simulink model "downlink_4c2t"  (Simulink 8.7)
settings: Solver=VariableStepDiscrete  StartTime=0.0  StopTime=DUC_LINEUP_param.endTime  RelTol=1e-3
PreLoadFcn:
  | % Run the setup script when the model is opened
  | setup_downlink_4c2t;
InitFcn:
  | % Run the setup script again just before the
  | % model is run, so that any updates made
  | % after opening are applied.
  | setup_downlink_4c2t;
  | 
  | %% DSPBuilder Start
  | alt_dspbuilder_update_model(bdroot)
  | %% DSPBuilder End
values from neighbouring files (symbols this model uses):
  LUTS_DPD_CLIP =     [downlink_4c2t_dpd_clip.mat]
  PulsExtention = 128    [setup_downlink_4c2t.m]
  StartAddress1 = Iter1_Param.BaseAddr + 3200    [setup_downlink_4c2t.m]
  StartAddress2 = StartAddress1+1024    [setup_downlink_4c2t.m]
  win = [w(1:PulsExtention) ones(1,Iter0_Param.pulseLen) w(PulsExtention+1:end)]    [setup_downlink_4c2t.m]
undefined symbols (not defined in the file or in its folder): AdvDSPBChannelOutDisplay, AdvDSPBDMemDisplay, dpoly, dspba_ChannelInVis, dspba_ChannelOutVis, dspba_internal_get_channel_ports, dspba_internal_get_demux_ports, DUC_LINEUP_param, evalAionMaskParam, iq_width, Iter0_Param, latency, primtype, REG, UseDontCare, value
undefined symbols (not defined in the file): cfr0_id, cfr_Params0, cfr_Params1, clock_rate, REG_dut_id_addr
libraries: DSPBAPrim x1438, DSPBAControl x77, DSPBAModelBus x71, DSPBABase x40, downlink_4c2t_foldingcfr_3firs_lib x26, DSPBAUtilities x8, downlink_4c2t_lib x4, downlink_4c2t_cordic_lib x2, downlink_4c2t_dpd_clipper x2, DSPBAFilters x2, DSPBAWaveformSynth x2, downlink_4c2t_lduc_lib x1
(part 1 of 17)
Description:
  | DSP Builder Advanced Template for Template Design implementing ModelIP designs
settings Model: Creator=mjervis  LastModifiedBy=5g
settings DataIOCC: SignalLoggingSaveFormat=ModelDataLogs
settings OptimizationCC: ExpressionDepthLimit=2147483647
settings DebuggingCC: SolverPrmCheckMsg=warning  InheritedTsInSrcMsg=none  IntegerOverflowMsg=none  FcnCallInpInsideContextMsg=UseLocalSettings  StateNameClashWarn=warning  IntegerSaturationMsg=none
settings GRTTargetCC: CombineOutputUpdateFcns=off  GRTInterface=on

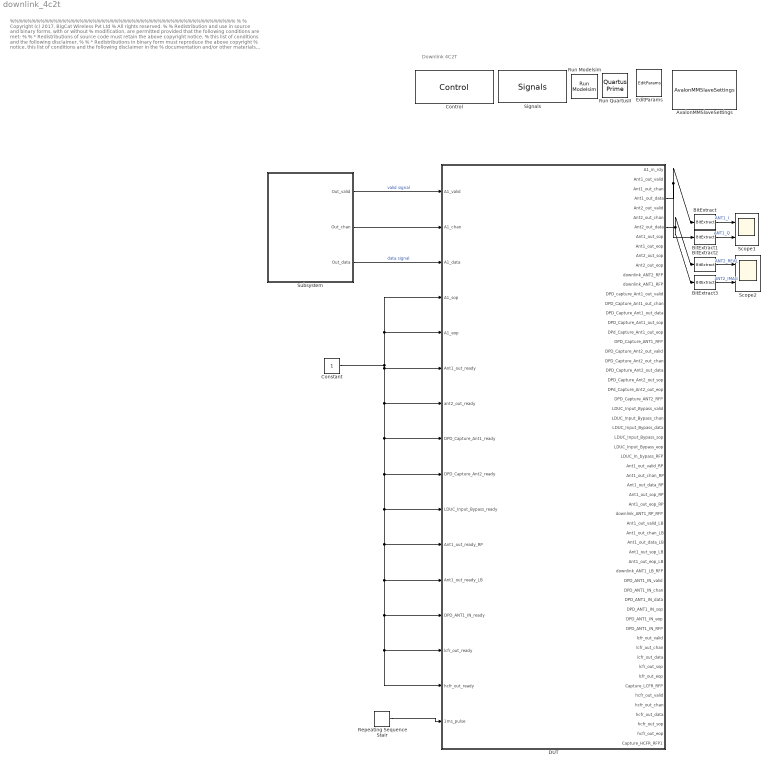
== system downlink_4c2t ==
  note: %%%%%%%%%%%%%%%%%%%%%%%%%%%%%%%%%%%%%%%%%%%%%%%%%%%%
      |  %
      |  % Copyright (c) 2017, BigCat Wireless Pvt Ltd
      |  % All rights reserved.
      |  %
      |  % Redistribution and use in source and binary forms, with or without
      |  % modification, are permitted provided that the following conditions are met:
      |  %
      |  %     * Redistributions of source code must retain the above copyright notice,
      |  %       this list of conditions and the following disclaimer.
      |  %
      |  %     * Redistributions in binary form must reproduce the above copyright
      |  %       notice, this list of conditions and the following disclaimer in the
      |  %       documentation and/or other materials provided with the distribution.
      |  %
      |  %     * Neither the name of the copyright holder nor the names of its contributors
      |  %       may be used to endorse or promote products derived from this software
      |  %       without specific prior written permission.
      |  %
      |  %
      |  %
      |  % THIS SOFTWARE IS PROVIDED BY THE COPYRIGHT HOLDERS AND CONTRIBUTORS "AS IS"
      |  % AND ANY EXPRESS OR IMPLIED WARRANTIES, INCLUDING, BUT NOT LIMITED TO, THE
      |  % IMPLIED WARRANTIES OF MERCHANTABILITY AND FITNESS FOR A PARTICULAR PURPOSE ARE
      |  % DISCLAIMED. IN NO EVENT SHALL THE COPYRIGHT HOLDER OR CONTRIBUTORS BE LIABLE
      |  % FOR ANY DIRECT, INDIRECT, INCIDENTAL, SPECIAL, EXEMPLARY, OR CONSEQUENTIAL
      |  % DAMAGES (INCLUDING, BUT NOT LIMITED TO, PROCUREMENT OF SUBSTITUTE GOODS OR
      |  % SERVICES; LOSS OF USE, DATA, OR PROFITS; OR BUSINESS INTERRUPTION) HOWEVER
      |  % CAUSED AND ON ANY THEORY OF LIABILITY, WHETHER IN CONTRACT, STRICT LIABILITY,
      |  % OR TORT (INCLUDING NEGLIGENCE OR OTHERWISE) ARISING IN ANY WAY OUT OF THE USE
      |  % OF THIS SOFTWARE, EVEN IF ADVISED OF THE POSSIBILITY OF SUCH DAMAGE.
      |  %
      |   %%%%%%%%%%%%%%%%%%%%%%%%%%%%%%%%%%%%%%%%%%%%%%%%%%%%%
  note: Downlink 4C2T
  AvalonMMSlaveSettings : DSPBABase/AvalonMMSlaveSettings
  BitExtract : DSPBAPrim/BitExtract  primtype=bitextract  nInputs=1  nOutputs=1  omode=Specify via dialog  otype=sfix(16)  scale=2^-15  rndmethod=Unbiased  factor=1  satmethod=Symmetric  shift_vec=[0 1 2 -1]  value=0  inPortNames=[' '; ' ';]  outPortNames=[' ']  dspbaimage=dspba_prim.jpg  text=fprintf('..%d', value);  style=Optimised  visibilities=8+1024  version=20090407
  BitExtract1 : DSPBAPrim/BitExtract  primtype=bitextract  nInputs=1  nOutputs=1  omode=Specify via dialog  otype=sfix(16)  scale=2^-15  rndmethod=Unbiased  factor=1  satmethod=Symmetric  shift_vec=[0 1 2 -1]  value=16  inPortNames=[' '; ' ';]  outPortNames=[' ']  dspbaimage=dspba_prim.jpg  text=fprintf('..%d', value);  style=Optimised  visibilities=8+1024  version=20090407
  BitExtract2 : DSPBAPrim/BitExtract  primtype=bitextract  nInputs=1  nOutputs=1  omode=Specify via dialog  otype=sfix(16)  scale=2^-15  rndmethod=Unbiased  factor=1  satmethod=Symmetric  shift_vec=[0 1 2 -1]  value=0  inPortNames=[' '; ' ';]  outPortNames=[' ']  dspbaimage=dspba_prim.jpg  text=fprintf('..%d', value);  style=Optimised  visibilities=8+1024  version=20090407
  BitExtract3 : DSPBAPrim/BitExtract  primtype=bitextract  nInputs=1  nOutputs=1  omode=Specify via dialog  otype=sfix(16)  scale=2^-15  rndmethod=Unbiased  factor=1  satmethod=Symmetric  shift_vec=[0 1 2 -1]  value=16  inPortNames=[' '; ' ';]  outPortNames=[' ']  dspbaimage=dspba_prim.jpg  text=fprintf('..%d', value);  style=Optimised  visibilities=8+1024  version=20090407
  Constant : Constant  OutDataTypeStr=boolean
  Control : DSPBABase/Control  generate=on  language=VHDL  destination=./rtl  destination_gui=./rtl  make_full_path=off  path_is_relative=on  autotestbench=off  signaldepth=2  coveragetestbench=off  logs=off  spacewidth=2  spacenum=1  addrwidth=14  datawidth=32  dataendian=Big Endian  hierarchicalnames=off  ramThresholdBits=-1  distRamThresholdBits=-1  mlabThresholdBits=-1  hardMultiplierThresholdLuts=-1  version=20090407  errorOnChanMismatch=1  errorOnGPIOMismatch=0  importModelsimResults=0  cycleAccurate=off  reinterpretCastMult=off  paramFile=downlink_4c2t_params.xml
  DUT : Subsystem
  EditParams : DSPBABase/EditParams  version=20090407
  Repeating Sequence Stair : simulink/Sources/Repeating Sequence Stair  OutValues=[zeros(1,1000) 1 1 1 1].'  tsamp=-1  OutMin=[]  OutMax=[]  OutDataTypeStr=fixdt('boolean')  OutputDataTypeScalingMode=Specify via dialog  OutDataType=fixdt('boolean')  ConRadixGroup=Best Precision: Vector-wise  OutScaling=[]
  Run Modelsim : DSPBABase/Run Modelsim  version=20090407
  "Run QuartusII " : DSPBABase/Quartus Prime  version=20090407
  Scope1 : Scope  NumInputPorts=2
  Scope2 : Scope  NumInputPorts=2
  Signals : DSPBABase/Signals  clk=clk  freq=DUC_LINEUP_param.ClockRate  margin=DUC_LINEUP_param.ClockMargin  rst=areset  rstactive=High  bus=bus  enbusclock=on  busfreq=61.44  bussync=on  version=20090407
  Subsystem : Subsystem
  wires:
  Subsystem/3(Out_data) -> DUT/3(A1_data)  "data signal"
  Subsystem/1(Out_valid) -> DUT/1(A1_valid)  "valid signal"
  Subsystem/2(Out_chan) -> DUT/2(A1_chan)
  Constant/1 -> DUT/8(DPD_Capture_Ant1_ready), DUT/9(DPD_Capture_Ant2_ready), DUT/10(LDUC_Input_Bypass_ready), DUT/11(Ant1_out_ready_RP), DUT/12(Ant1_out_ready_LB), DUT/14(lcfr_out_ready), DUT/15(hcfr_out_ready), DUT/13(DPD_ANT1_IN_ready), DUT/7(ant2_out_ready), DUT/6(Ant1_out_ready), DUT/4(A1_sop), DUT/5(A1_eop)
  DUT/7(Ant2_out_data) -> BitExtract2/1, BitExtract3/1
  BitExtract/1 -> Scope1/1  "ANT1_I"
  BitExtract1/1 -> Scope1/2  "ANT1_Q"
  BitExtract2/1 -> Scope2/1  "ANT2_REAL"
  BitExtract3/1 -> Scope2/2  "ANT2_IMAG"
  Repeating Sequence Stair/1 -> DUT/16(1ms_pulse)
  DUT/4(Ant1_out_data) -> BitExtract1/1, BitExtract/1

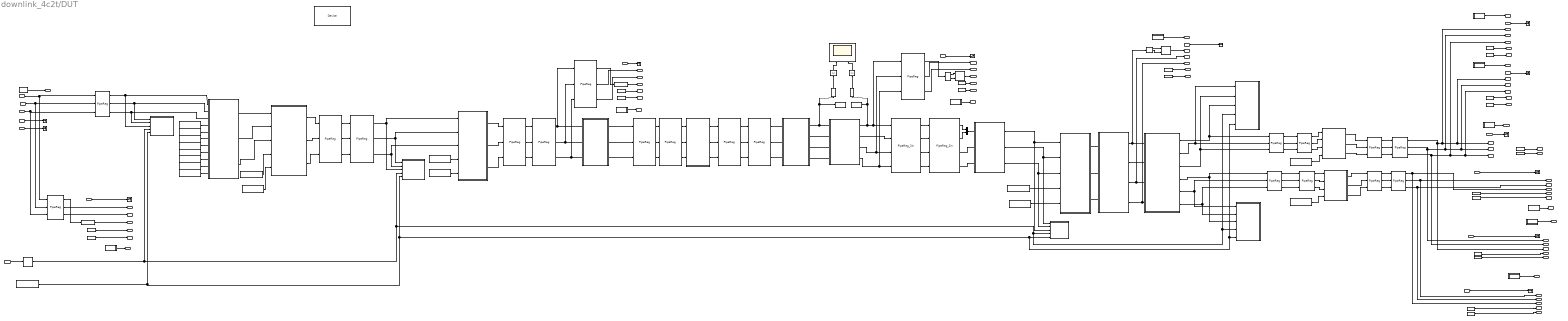
== system downlink_4c2t/DUT ==
  A1_valid : Inport
  A1_chan : Inport  Port=2
  A1_data : Inport  Port=3
  A1_sop : Inport  Port=4
  A1_eop : Inport  Port=5
  Ant1_out_ready : Inport  Port=6
  ant2_out_ready : Inport  Port=7
  DPD_Capture_Ant1_ready : Inport  Port=8
  DPD_Capture_Ant2_ready : Inport  Port=9
  LDUC_Input_Bypass_ready : Inport  Port=10
  Ant1_out_ready_RP : Inport  Port=11
  Ant1_out_ready_LB : Inport  Port=12
  DPD_ANT1_IN_ready : Inport  Port=13
  lcfr_out_ready : Inport  Port=14
  hcfr_out_ready : Inport  Port=15
  1ms_pulse : Inport  Port=16
  ANT1_rfp : Subsystem
  ANT2_rfp : Subsystem
  Abs2 : Abs
  Abs3 : Abs
  BLIND_CFR : Subsystem
  BitCombine : DSPBAPrim/BitCombine  primtype=bitcombine  nInputs=2  nOutputs=1  omode=Inherit via internal rule  otype=sfix(16)  scale=2^-15  rndmethod=Unbiased  factor=1  satmethod=Symmetric  shift_vec=[0 1 2 -1]  value=0  inPortNames=['l'; 'h';]  outPortNames=[' ']  dspbaimage=dspba_prim.jpg  text=fprintf('[h,l]');  style=Optimised  visibilities=8+2  version=20090407
  BitCombine1 : DSPBAPrim/BitCombine  primtype=bitcombine  nInputs=2  nOutputs=1  omode=Inherit via internal rule  otype=sfix(16)  scale=2^-15  rndmethod=Unbiased  factor=1  satmethod=Symmetric  shift_vec=[0 1 2 -1]  value=0  inPortNames=['l'; 'h';]  outPortNames=[' ']  dspbaimage=dspba_prim.jpg  text=fprintf('[h,l]');  style=Optimised  visibilities=8+2  version=20090407
  COMPLEX_REAL : Subsystem
  Complex to Real-Imag : ComplexToRealImag
  Complex to Real-Imag1 : ComplexToRealImag
  Const1 : DSPBAPrim/Const  primtype=const  nInputs=0  nOutputs=1  omode=boolean  otype=sfix(16)  scale=2^-15  rndmethod=Unbiased  factor=1  satmethod=Symmetric  shift_vec=[0 1 2 -1]  value=1  inPortNames=['+'; '+';]  outPortNames=[' ']  dspbaimage=dspba_prim.jpg  text=fprintf('%s', num2str(value));  style=Optimised  visibilities=8 + 1024  floatPrecision=float32_m23  version=20120820
  Const{2..17,19,30} (18 alike) : DSPBAPrim/Const  primtype=const  nInputs=0  nOutputs=1  omode=Inherit via internal rule  otype=sfix(16)  scale=2^-15  rndmethod=Unbiased  factor=1  satmethod=Symmetric  shift_vec=[0 1 2 -1]  value=1  inPortNames=['+'; '+';]  outPortNames=[' ']  dspbaimage=dspba_prim.jpg  text=fprintf('%s', num2str(value));  style=Optimised  visibilities=8 + 1024  floatPrecision=float32_m23  version=20120820
  Const18 : DSPBAPrim/Const  primtype=const  nInputs=0  nOutputs=1  omode=boolean  otype=sfix(16)  scale=2^-15  rndmethod=Unbiased  factor=1  satmethod=Symmetric  shift_vec=[0 1 2 -1]  value=1  inPortNames=['+'; '+';]  outPortNames=[' ']  dspbaimage=dspba_prim.jpg  text=fprintf('%s', num2str(value));  style=Optimised  visibilities=8 + 1024  floatPrecision=float32_m23  version=20120820
  Const29 : DSPBAPrim/Const  primtype=const  nInputs=0  nOutputs=1  omode=boolean  otype=sfix(16)  scale=2^-15  rndmethod=Unbiased  factor=1  satmethod=Symmetric  shift_vec=[0 1 2 -1]  value=1  inPortNames=['+'; '+';]  outPortNames=[' ']  dspbaimage=dspba_prim.jpg  text=fprintf('%s', num2str(value));  style=Optimised  visibilities=8 + 1024  floatPrecision=float32_m23  version=20120820
  Convert1 : DSPBAPrim/Convert  primtype=convert  nInputs=1  nOutputs=1  omode=Specify via dialog  otype=sfix(32)  scale=2^-31  rndmethod=Unbiased  factor=1  satmethod=None  shift_vec=[0 1 2 -1]  value=round([0:255]/17)  inPortNames=[' '; ' ';]  outPortNames=[' '; 'c']  dspbaimage=dspba_prim.jpg  text=fprintf('convert');  style=Optimised  visibilities=8+64+256+2^17  clipdetect=off  floatPrecision=float32_m23  advOptions=[]  version=20130211
  Convert2 : DSPBAPrim/Convert  primtype=convert  nInputs=1  nOutputs=1  omode=Specify via dialog  otype=sfix(32)  scale=2^-31  rndmethod=Unbiased  factor=1  satmethod=None  shift_vec=[0 1 2 -1]  value=round([0:255]/17)  inPortNames=[' '; ' ';]  outPortNames=[' '; 'c']  dspbaimage=dspba_prim.jpg  text=fprintf('convert');  style=Optimised  visibilities=8+64+256+2^17  clipdetect=off  floatPrecision=float32_m23  advOptions=[]  version=20130211
  DPD : Subsystem
  DPD1_CLIPPER : Subsystem
  DPD2_CLIPPER : Subsystem
  DPD_ANT1_IN_rfp : Subsystem
  DUC_DPD1_OUT_PM : Subsystem
  DUC_DPD2_OUT_PM : Subsystem
  DUC_DPD_IN_PM : Subsystem
  DUC_IN_PM : Subsystem
  DUC_SUMMER_PM : Subsystem
  Data Type Conversion2 : DataTypeConversion  OutDataTypeStr=double
  Data Type Conversion4 : DataTypeConversion  OutDataTypeStr=double
  Device : DSPBABase/Device  family=Arria 10  deviceMember=Arria 10  stratix4device=Stratix IV GX  hardcopy4device=HardCopy IV E  stratix5device=Stratix V GX  device=10AS066N3F40E2SGE2  speed=2  stratixSpeed=-5  stratix2Speed=-3  stratix3Speed=-3  stratix4gxSpeed=-2  stratix4gtSpeed=-1  cyclone2Speed=-6  cyclone3Speed=-7  arria2Speed=-4  cyclone4eSpeed=-8  stratix5Speed=-3  arria5Speed=-4  arriaSpeed=-6  cyclone3lsSpeed=-7  cyclone5Speed=-6  arria2gzSpeed=-3  nightFurySpeed=-2  ecp2Speed=-7  hardcopycompat=off  version=20140217  max10flashmode=off  max10nomeminit=off
  Downlink_ANT1_LB_rfp : Subsystem
  Downlink_ANT1_RP_rfp : Subsystem
  Gain_dpd_input : Subsystem
  Gain_duc_input : Subsystem
  Gain_summer : Subsystem
  HDUC_STG1 : Subsystem
  HDUC_STG2 : Subsystem
  LDUC : Subsystem
  Mux : Mux  Inputs=2
  PipeReg_2in : downlink_4c2t_foldingcfr_3firs_lib/PipeReg_2in  NPipe=2  Clock_Margin=DUC_LINEUP_param.ClockMargin
      link override ChannelOut: value=2  packetBeginEnabled=off  latency=2
  PipeReg_2in1 : downlink_4c2t_foldingcfr_3firs_lib/PipeReg_2in  NPipe=2  Clock_Margin=DUC_LINEUP_param.ClockMargin
      link override ChannelOut: value=2  packetBeginEnabled=off  latency=2
  PipeReg_CM_HDUC_R1 : downlink_4c2t_foldingcfr_3firs_lib/PipeReg  NPipe=2  Clock_Margin=DUC_LINEUP_param.ClockMargin
      link override ChannelOut: latency=2  value=1  packetBeginEnabled=off
  PipeReg_HDCU2_RC1 : downlink_4c2t_foldingcfr_3firs_lib/PipeReg  NPipe=2  Clock_Margin=DUC_LINEUP_param.ClockMargin
      link override ChannelOut: latency=2  value=1  packetBeginEnabled=off
  PipeReg_HDCU2_RC_L1 : downlink_4c2t_foldingcfr_3firs_lib/PipeReg  NPipe=2  Clock_Margin=DUC_LINEUP_param.ClockMargin
      link override ChannelOut: latency=2  value=1  packetBeginEnabled=off
  PipeReg_HDUC2_RC_L1 : downlink_4c2t_foldingcfr_3firs_lib/PipeReg  NPipe=2  Clock_Margin=DUC_LINEUP_param.ClockMargin
      link override ChannelOut: latency=2  value=1  packetBeginEnabled=off
  PipeReg_HDUC_RC_L : downlink_4c2t_foldingcfr_3firs_lib/PipeReg  NPipe=2  Clock_Margin=DUC_LINEUP_param.ClockMargin
      link override ChannelOut: value=1  packetBeginEnabled=off  latency=2
  PipeReg_HDUC_RC_R : downlink_4c2t_foldingcfr_3firs_lib/PipeReg  NPipe=2  Clock_Margin=DUC_LINEUP_param.ClockMargin
      link override ChannelOut: latency=2  value=1  packetBeginEnabled=off
  PipeReg_avln_avln_R : downlink_4c2t_foldingcfr_3firs_lib/PipeReg  NPipe=6  Clock_Margin=DUC_LINEUP_param.ClockMargin
      link override ChannelOut: latency=6  value=1  packetBeginEnabled=off
  PipeReg_dpd1clip_avln_L : downlink_4c2t_foldingcfr_3firs_lib/PipeReg  NPipe=2  Clock_Margin=DUC_LINEUP_param.ClockMargin
      link override ChannelOut: latency=2  value=1  packetBeginEnabled=off
  PipeReg_dpd1clip_avln_R : downlink_4c2t_foldingcfr_3firs_lib/PipeReg  NPipe=2  Clock_Margin=DUC_LINEUP_param.ClockMargin
      link override ChannelOut: latency=2  value=1  packetBeginEnabled=off
  PipeReg_dpd1gain_dpd1clip_L : downlink_4c2t_foldingcfr_3firs_lib/PipeReg  NPipe=2  Clock_Margin=DUC_LINEUP_param.ClockMargin
      link override ChannelOut: latency=2  value=1  packetBeginEnabled=off
  PipeReg_dpd1gain_dpd1clip_R : downlink_4c2t_foldingcfr_3firs_lib/PipeReg  NPipe=2  Clock_Margin=DUC_LINEUP_param.ClockMargin
      link override ChannelOut: latency=2  value=1  packetBeginEnabled=off
  PipeReg_dpd2clip_avln_L : downlink_4c2t_foldingcfr_3firs_lib/PipeReg  NPipe=2  Clock_Margin=DUC_LINEUP_param.ClockMargin
      link override ChannelOut: latency=2  value=1  packetBeginEnabled=off
  PipeReg_dpd2clip_avln_R : downlink_4c2t_foldingcfr_3firs_lib/PipeReg  NPipe=2  Clock_Margin=DUC_LINEUP_param.ClockMargin
      link override ChannelOut: latency=2  value=1  packetBeginEnabled=off
  PipeReg_dpd2gain_dpd2clip_L : downlink_4c2t_foldingcfr_3firs_lib/PipeReg  NPipe=2  Clock_Margin=DUC_LINEUP_param.ClockMargin
      link override ChannelOut: latency=2  value=1  packetBeginEnabled=off
  PipeReg_dpd2gain_dpd2clip_R : downlink_4c2t_foldingcfr_3firs_lib/PipeReg  NPipe=2  Clock_Margin=DUC_LINEUP_param.ClockMargin
      link override ChannelOut: latency=2  value=1  packetBeginEnabled=off
  PipeReg_lduc_RC_L : downlink_4c2t_foldingcfr_3firs_lib/PipeReg  NPipe=2  Clock_Margin=DUC_LINEUP_param.ClockMargin
      link override ChannelOut: latency=2  value=1  packetBeginEnabled=off
  PipeReg_lduc_RC_R : downlink_4c2t_foldingcfr_3firs_lib/PipeReg  NPipe=2  Clock_Margin=DUC_LINEUP_param.ClockMargin
      link override ChannelOut: latency=2  value=1  packetBeginEnabled=off
  PipeReg_lduc_hduc1_L : downlink_4c2t_foldingcfr_3firs_lib/PipeReg  NPipe=2  Clock_Margin=DUC_LINEUP_param.ClockMargin
      link override ChannelOut: latency=2  value=1  packetBeginEnabled=off
  PipeReg_lduc_hduc1_L2 : downlink_4c2t_foldingcfr_3firs_lib/PipeReg  NPipe=6  Clock_Margin=DUC_LINEUP_param.ClockMargin
      link override ChannelOut: latency=6  value=1  packetBeginEnabled=off
  PipeReg_lduc_hduc1_R : downlink_4c2t_foldingcfr_3firs_lib/PipeReg  NPipe=2  Clock_Margin=DUC_LINEUP_param.ClockMargin
      link override ChannelOut: latency=2  value=1  packetBeginEnabled=off
  REAL_COMPLEX1 : Subsystem
  REAL_COMPLEX2 : Subsystem
  RegBit : DSPBAModelBus/RegBit  reg_name=Reg_busy_bit_addr  reg_rwmode=Read/Write  reg_lsb=0  reg_init=0  reg_desc=Reg_busy_bi will be stored here  reg_addr=9686  reg_desc0=0  reg_desc1=0  SampleTime=-1  version=20090407
  RegBit1 : DSPBAModelBus/RegBit  reg_name=DUC_LINEUP_param.A12xC_NCO.Sync  reg_rwmode=Read/Write  reg_lsb=0  reg_init=0  reg_desc=Description of what is stored in this field  reg_addr=768  reg_desc0=0  reg_desc1=0  SampleTime=1  version=20090407
  RegField : DSPBAModelBus/RegField  reg_name=Sum_shifter_addr  reg_rwmode=Read/Write  reg_msb=1  reg_lsb=0  reg_mode=Specify via dialog  reg_type=uint(2)  reg_scale=2^-0  reg_init=Sum_shifter_init_value  reg_desc=Sum_shifter_init_value will be stored  reg_modal=off  reg_desc0=0  reg_desc1=0  reg_desc2=0  reg_desc3=0  reg_desc4=0  reg_desc5=0  reg_desc6=0  reg_desc7=0  reg_addr=9643  SampleTime=-1  version=20090407
  RegField1 : DSPBAModelBus/RegField  reg_name=DPD1_CLIP_SCALE  reg_rwmode=Read/Write  reg_msb=0  reg_lsb=0  reg_mode=Specify via dialog  reg_type=ufix(1)  reg_scale=1  reg_init=DPD1_CLIP_INIT_VALUE  reg_desc=DPD1_CLIP_INIT_VALUE will be stored  reg_modal=off  reg_desc0=0  reg_desc1=0  reg_desc2=0  reg_desc3=0  reg_desc4=0  reg_desc5=0  reg_desc6=0  reg_desc7=0  reg_addr=9691  SampleTime=-1  version=20090407
  RegField10 : DSPBAModelBus/RegField  reg_name=ant1_summer_gain_addr  reg_rwmode=Read/Write  reg_msb=15  reg_lsb=0  reg_mode=Specify via dialog  reg_type=ufix(16)  reg_scale=2^-12  reg_init=ant1_summer_gain_init  reg_desc=ant1_summer_gain will be stored here  reg_modal=off  reg_desc0=0  reg_desc1=0  reg_desc2=0  reg_desc3=0  reg_desc4=0  reg_desc5=0  reg_desc6=0  reg_desc7=0  reg_addr=9624  SampleTime=-1  version=20090407
  RegField11 : DSPBAModelBus/RegField  reg_name=ant2_summer_gain_addr  reg_rwmode=Read/Write  reg_msb=15  reg_lsb=0  reg_mode=Specify via dialog  reg_type=ufix(16)  reg_scale=2^-12  reg_init=ant2_summer_gain_init  reg_desc=ant2_summer_gain will be stored here  reg_modal=off  reg_desc0=0  reg_desc1=0  reg_desc2=0  reg_desc3=0  reg_desc4=0  reg_desc5=0  reg_desc6=0  reg_desc7=0  reg_addr=9625  SampleTime=-1  version=20090407
  RegField12 : DSPBAModelBus/RegField  reg_name=dpd1_gain_addr  reg_rwmode=Read/Write  reg_msb=15  reg_lsb=0  reg_mode=Specify via dialog  reg_type=ufix(16)  reg_scale=2^-12  reg_init=dpd1_gain_init_value  reg_desc=dpd1_gain will be stored here  reg_modal=off  reg_desc0=0  reg_desc1=0  reg_desc2=0  reg_desc3=0  reg_desc4=0  reg_desc5=0  reg_desc6=0  reg_desc7=0  reg_addr=9626  SampleTime=-1  version=20090407
  RegField13 : DSPBAModelBus/RegField  reg_name=dpd2_gain_addr  reg_rwmode=Read/Write  reg_msb=15  reg_lsb=0  reg_mode=Specify via dialog  reg_type=ufix(16)  reg_scale=2^-12  reg_init=dpd2_gain_init_value  reg_desc=dpd2_gain will be stored here  reg_modal=off  reg_desc0=0  reg_desc1=0  reg_desc2=0  reg_desc3=0  reg_desc4=0  reg_desc5=0  reg_desc6=0  reg_desc7=0  reg_addr=9627  SampleTime=-1  version=20090407
  RegField14 : DSPBAModelBus/RegField  reg_name=DPD2_CLIP_SCALE  reg_rwmode=Read/Write  reg_msb=0  reg_lsb=0  reg_mode=Specify via dialog  reg_type=ufix(1)  reg_scale=1  reg_init=DPD2_CLIP_INIT_VALUE  reg_desc=DPD2_CLIP_INIT_VALUE will be stored  reg_modal=off  reg_desc0=0  reg_desc1=0  reg_desc2=0  reg_desc3=0  reg_desc4=0  reg_desc5=0  reg_desc6=0  reg_desc7=0  reg_addr=9692  SampleTime=-1  version=20090407
  RegField2 : DSPBAModelBus/RegField  reg_name=ant1_carr1_gain_addr  reg_rwmode=Read/Write  reg_msb=15  reg_lsb=0  reg_mode=Specify via dialog  reg_type=ufix(16)  reg_scale=2^-12  reg_init=ant1_carr1_gain_val_init  reg_desc=ant1_carr1_gain will be stored here  reg_modal=off  reg_desc0=0  reg_desc1=0  reg_desc2=0  reg_desc3=0  reg_desc4=0  reg_desc5=0  reg_desc6=0  reg_desc7=0  reg_addr=9616  SampleTime=-1  version=20090407
  RegField3 : DSPBAModelBus/RegField  reg_name=ant1_carr2_gain_addr  reg_rwmode=Read/Write  reg_msb=15  reg_lsb=0  reg_mode=Specify via dialog  reg_type=ufix(16)  reg_scale=2^-12  reg_init=ant1_carr2_gain_val_init  reg_desc=ant1_carr2_gain will be stored here  reg_modal=off  reg_desc0=0  reg_desc1=0  reg_desc2=0  reg_desc3=0  reg_desc4=0  reg_desc5=0  reg_desc6=0  reg_desc7=0  reg_addr=9617  SampleTime=-1  version=20090407
  RegField4 : DSPBAModelBus/RegField  reg_name=ant1_carr3_gain_addr  reg_rwmode=Read/Write  reg_msb=15  reg_lsb=0  reg_mode=Specify via dialog  reg_type=ufix(16)  reg_scale=2^-12  reg_init=ant1_carr3_gain_val_init  reg_desc=ant1_carr3_gain will be stored here  reg_modal=off  reg_desc0=0  reg_desc1=0  reg_desc2=0  reg_desc3=0  reg_desc4=0  reg_desc5=0  reg_desc6=0  reg_desc7=0  reg_addr=9618  SampleTime=-1  version=20090407
  RegField5 : DSPBAModelBus/RegField  reg_name=ant1_carr4_gain_addr  reg_rwmode=Read/Write  reg_msb=15  reg_lsb=0  reg_mode=Specify via dialog  reg_type=ufix(16)  reg_scale=2^-12  reg_init=ant1_carr4_gain_val_init  reg_desc=ant1_carr4_gain will be stored here  reg_modal=off  reg_desc0=0  reg_desc1=0  reg_desc2=0  reg_desc3=0  reg_desc4=0  reg_desc5=0  reg_desc6=0  reg_desc7=0  reg_addr=9619  SampleTime=-1  version=20090407
  RegField6 : DSPBAModelBus/RegField  reg_name=ant2_carr1_gain_addr  reg_rwmode=Read/Write  reg_msb=15  reg_lsb=0  reg_mode=Specify via dialog  reg_type=ufix(16)  reg_scale=2^-12  reg_init=ant2_carr1_gain_val_init  reg_desc=ant2_carr1_gain will be stored here  reg_modal=off  reg_desc0=0  reg_desc1=0  reg_desc2=0  reg_desc3=0  reg_desc4=0  reg_desc5=0  reg_desc6=0  reg_desc7=0  reg_addr=9620  SampleTime=-1  version=20090407
  RegField7 : DSPBAModelBus/RegField  reg_name=ant2_carr2_gain_addr  reg_rwmode=Read/Write  reg_msb=15  reg_lsb=0  reg_mode=Specify via dialog  reg_type=ufix(16)  reg_scale=2^-12  reg_init=ant2_carr2_gain_val_init  reg_desc=ant2_carr2_gain will be stored here  reg_modal=off  reg_desc0=0  reg_desc1=0  reg_desc2=0  reg_desc3=0  reg_desc4=0  reg_desc5=0  reg_desc6=0  reg_desc7=0  reg_addr=9621  SampleTime=-1  version=20090407
  RegField8 : DSPBAModelBus/RegField  reg_name=ant2_carr3_gain_addr  reg_rwmode=Read/Write  reg_msb=15  reg_lsb=0  reg_mode=Specify via dialog  reg_type=ufix(16)  reg_scale=2^-12  reg_init=ant2_carr3_gain_val_init  reg_desc=ant2_carr3_gain will be stored here  reg_modal=off  reg_desc0=0  reg_desc1=0  reg_desc2=0  reg_desc3=0  reg_desc4=0  reg_desc5=0  reg_desc6=0  reg_desc7=0  reg_addr=9622  SampleTime=-1  version=20090407
  RegField9 : DSPBAModelBus/RegField  reg_name=ant2_carr4_gain_addr  reg_rwmode=Read/Write  reg_msb=15  reg_lsb=0  reg_mode=Specify via dialog  reg_type=ufix(16)  reg_scale=2^-12  reg_init=ant2_carr4_gain_val_init  reg_desc=ant2_carr4_gain will be stored here  reg_modal=off  reg_desc0=0  reg_desc1=0  reg_desc2=0  reg_desc3=0  reg_desc4=0  reg_desc5=0  reg_desc6=0  reg_desc7=0  reg_addr=9623  SampleTime=-1  version=20090407
  SampleDelay : DSPBAPrim/SampleDelay  primtype=sampdelay  nInputs=1  nOutputs=1  omode=Inherit via internal rule  otype=sfix(16)  scale=2^-15  rndmethod=Unbiased  factor=1  satmethod=Symmetric  shift_vec=[0 1 2 -1]  value=4  inPortNames=[' '; ' ';]  outPortNames=[' ']  dspbaimage=dspba_prim.jpg  text=dpoly(1, eye(1,value+1), 'z')  style=Optimised  visibilities=8 + 1024 + 2^17 + 2^18  flexible=off  slackgroup=0  augmented=0  version=20090407  advOptions=[]
  Scope1 : Scope  NumInputPorts=2
  Terminator{1..10,19..20} (12 alike) : Terminator
  To Workspace1 : ToWorkspace  VariableName=cfr_input  SaveFormat=Structure With Time  SampleTime=1
  To Workspace3 : ToWorkspace  VariableName=cfr_output  SaveFormat=Structure With Time  SampleTime=1
  dpd_ant1_out_rfp : Subsystem
  dpd_ant2_out_rfp : Subsystem
  lcfr_rfp : Subsystem
  lcfr_rfp1 : Subsystem
  lduc_bypass_rfp : Subsystem
  A1_in_rdy : Outport
  Ant1_out_valid : Outport  Port=2
  Ant1_out_chan : Outport  Port=3
  Ant1_out_data : Outport  Port=4
  Ant2_out_valid : Outport  Port=5
  Ant2_out_chan : Outport  Port=6
  Ant2_out_data : Outport  Port=7
  Ant1_out_sop : Outport  Port=8
  Ant1_out_eop : Outport  Port=9
  Ant2_out_sop : Outport  Port=10
  Ant2_out_eop : Outport  Port=11
  downlink_ANT2_RFP : Outport  Port=12
  downlink_ANT1_RFP : Outport  Port=13
  DPD_capture_Ant1_out_valid : Outport  Port=14
  DPD_Capture_Ant1_out_chan : Outport  Port=15
  DPD_Capture_Ant1_out_data : Outport  Port=16
  DPD_Capture_Ant1_out_sop : Outport  Port=17
  DPd_Capture_Ant1_out_eop : Outport  Port=18
  DPD_Capture_ANT1_RFP : Outport  Port=19
  DPD_Capture_Ant2_out_valid : Outport  Port=20
  DPD_Capture_Ant2_out_chan : Outport  Port=21
  DPD_Capture_Ant2_out_data : Outport  Port=22
  DPD_Capture_Ant2_out_sop : Outport  Port=23
  DPd_Capture_Ant2_out_eop : Outport  Port=24
  DPD_Capture_ANT2_RFP : Outport  Port=25
  LDUC_Input_Bypass_valid : Outport  Port=26
  LDUC_Input_Bypass_chan : Outport  Port=27
  LDUC_Input_Bypass_data : Outport  Port=28
  LDUC_Input_Bypass_sop : Outport  Port=29
  LDUC_Input_Bypass_eop : Outport  Port=30
  LDUC_In_bypass_RFP : Outport  Port=31
  Ant1_out_valid_RP : Outport  Port=32
  Ant1_out_chan_RP : Outport  Port=33
  Ant1_out_data_RP : Outport  Port=34
  Ant1_out_sop_RP : Outport  Port=35
  Ant1_out_eop_RP : Outport  Port=36
  downlink_ANT1_RP_RFP : Outport  Port=37
  Ant1_out_valid_LB : Outport  Port=38
  Ant1_out_chan_LB : Outport  Port=39
  Ant1_out_data_LB : Outport  Port=40
  Ant1_out_sop_LB : Outport  Port=41
  Ant1_out_eop_LB : Outport  Port=42
  downlink_ANT1_LB_RFP : Outport  Port=43
  DPD_ANT1_IN_valid : Outport  Port=44
  DPD_ANT1_IN_chan : Outport  Port=45
  DPD_ANT1_IN_data : Outport  Port=46
  DPD_ANT1_IN_sop : Outport  Port=47
  DPD_ANT1_IN_eop : Outport  Port=48
  DPD_ANT1_IN_RFP : Outport  Port=49
  lcfr_out_valid : Outport  Port=50
  lcfr_out_chan : Outport  Port=51
  lcfr_out_data : Outport  Port=52
  lcfr_out_sop : Outport  Port=53
  lcfr_out_eop : Outport  Port=54
  Capture_LCFR_RFP : Outport  Port=55
  hcfr_out_valid : Outport  Port=56
  hcfr_out_chan : Outport  Port=57
  hcfr_out_data : Outport  Port=58
  hcfr_out_sop : Outport  Port=59
  hcfr_out_eop : Outport  Port=60
  Capture_HCFR_RFP1 : Outport  Port=61
  wires:
  A1_sop/1 -> Terminator7/1
  A1_eop/1 -> Terminator8/1
  Const1/1 -> A1_in_rdy/1
  Const3/1 -> Ant1_out_sop/1
  Const5/1 -> Ant1_out_eop/1
  Ant1_out_ready/1 -> Terminator19/1
  PipeReg_dpd2clip_avln_R/2 -> DPD_Capture_Ant2_out_valid/1, Ant2_out_valid/1
  PipeReg_dpd2clip_avln_R/3 -> DPD_Capture_Ant2_out_chan/1, Ant2_out_chan/1
  PipeReg_dpd2clip_avln_R/1 -> DPD_Capture_Ant2_out_data/1, Ant2_out_data/1
  Const8/1 -> Ant2_out_sop/1
  Const9/1 -> Ant2_out_eop/1
  ant2_out_ready/1 -> Terminator20/1
  ANT2_rfp/1(Out_RFP) -> downlink_ANT2_RFP/1
  ANT1_rfp/1(Out_RFP) -> downlink_ANT1_RFP/1
  PipeReg_dpd1clip_avln_R/2 -> DPD_capture_Ant1_out_valid/1, Ant1_out_valid_RP/1, Ant1_out_valid_LB/1, Ant1_out_valid/1
  PipeReg_dpd1clip_avln_R/3 -> DPD_Capture_Ant1_out_chan/1, Ant1_out_chan_RP/1, Ant1_out_chan_LB/1, Ant1_out_chan/1
  Const2/1 -> DPD_Capture_Ant1_out_sop/1
  Const7/1 -> DPd_Capture_Ant1_out_eop/1
  DPD_Capture_Ant1_ready/1 -> Terminator2/1
  dpd_ant1_out_rfp/1(Out_RFP) -> DPD_Capture_ANT1_RFP/1
  Const10/1 -> DPD_Capture_Ant2_out_sop/1
  Const11/1 -> DPd_Capture_Ant2_out_eop/1
  DPD_Capture_Ant2_ready/1 -> Terminator3/1
  dpd_ant2_out_rfp/1(Out_RFP) -> DPD_Capture_ANT2_RFP/1
  PipeReg_avln_avln_R/2 -> LDUC_Input_Bypass_valid/1
  PipeReg_avln_avln_R/3 -> LDUC_Input_Bypass_chan/1
  Convert1/1 -> LDUC_Input_Bypass_data/1
  Const4/1 -> LDUC_Input_Bypass_sop/1
  Const6/1 -> LDUC_Input_Bypass_eop/1
  LDUC_Input_Bypass_ready/1 -> Terminator1/1
  lduc_bypass_rfp/1(Out_RFP) -> LDUC_In_bypass_RFP/1
  PipeReg_lduc_RC_L/1 -> PipeReg_lduc_RC_R/1
  PipeReg_lduc_RC_L/2 -> PipeReg_lduc_RC_R/2
  PipeReg_lduc_RC_L/3 -> PipeReg_lduc_RC_R/3
  RegBit1/1 -> LDUC/4(In_sync_pulse)
  LDUC/1(Out1) -> PipeReg_lduc_RC_L/1
  PipeReg_avln_avln_R/1 -> Convert1/1
  Const12/1 -> Ant1_out_sop_RP/1
  Const13/1 -> Ant1_out_eop_RP/1
  Ant1_out_ready_RP/1 -> Terminator4/1
  Downlink_ANT1_RP_rfp/1(Out_RFP) -> downlink_ANT1_RP_RFP/1
  PipeReg_dpd1clip_avln_R/1 -> DPD_Capture_Ant1_out_data/1, Ant1_out_data_RP/1, Ant1_out_data_LB/1, Ant1_out_data/1
  Const14/1 -> Ant1_out_sop_LB/1
  Const15/1 -> Ant1_out_eop_LB/1
  Ant1_out_ready_LB/1 -> Terminator5/1
  Downlink_ANT1_LB_rfp/1(Out_RFP) -> downlink_ANT1_LB_RFP/1
  Const16/1 -> DPD_ANT1_IN_sop/1
  Const17/1 -> DPD_ANT1_IN_eop/1
  DPD_ANT1_IN_ready/1 -> Terminator9/1
  DPD_ANT1_IN_rfp/1(Out_RFP) -> DPD_ANT1_IN_RFP/1
  Complex to Real-Imag/1 -> BitCombine/1
  Complex to Real-Imag/2 -> BitCombine/2
  BitCombine/1 -> DPD_ANT1_IN_data/1
  PipeReg_HDUC_RC_L/3 -> PipeReg_HDUC_RC_R/3
  PipeReg_HDUC_RC_L/2 -> PipeReg_HDUC_RC_R/2
  PipeReg_HDUC_RC_L/1 -> PipeReg_HDUC_RC_R/1
  HDUC_STG1/3(qc) -> PipeReg_HDUC_RC_L/3
  PipeReg_HDUC_RC_R/1 -> HDUC_STG2/1(a1)
  PipeReg_HDUC_RC_R/2 -> HDUC_STG2/2(v)
  PipeReg_HDUC_RC_R/3 -> HDUC_STG2/3(c)
  PipeReg_lduc_hduc1_R/1 -> PipeReg_CM_HDUC_R1/1, HDUC_STG1/1(a1)
  PipeReg_lduc_hduc1_R/2 -> PipeReg_CM_HDUC_R1/2, HDUC_STG1/2(v)
  PipeReg_lduc_hduc1_R/3 -> PipeReg_CM_HDUC_R1/3, HDUC_STG1/3(c)
  lcfr_rfp/1(Out_RFP) -> Capture_LCFR_RFP/1
  LDUC/2(Out2) -> PipeReg_lduc_RC_L/2
  HDUC_STG1/1(q1) -> PipeReg_HDUC_RC_L/1
  HDUC_STG1/2(qv) -> PipeReg_HDUC_RC_L/2
  BitCombine1/1 -> hcfr_out_data/1
  hcfr_out_ready/1 -> Terminator10/1
  Const18/1 -> hcfr_out_sop/1
  Const19/1 -> hcfr_out_eop/1
  lcfr_rfp1/1(Out_RFP) -> Capture_HCFR_RFP1/1
  Const29/1 -> lcfr_out_sop/1
  Const30/1 -> lcfr_out_eop/1
  Convert2/1 -> lcfr_out_data/1
  PipeReg_CM_HDUC_R1/1 -> Convert2/1
  PipeReg_CM_HDUC_R1/2 -> lcfr_out_valid/1
  PipeReg_CM_HDUC_R1/3 -> lcfr_out_chan/1
  lcfr_out_ready/1 -> Terminator6/1
  PipeReg_HDUC2_RC_L1/2 -> hcfr_out_valid/1
  PipeReg_HDUC2_RC_L1/3 -> hcfr_out_chan/1
  RegField2/1 -> Gain_duc_input/4(carr1_gain_val)
  RegField3/1 -> Gain_duc_input/5(carr2_gain_val)
  RegField4/1 -> Gain_duc_input/6(carr3_gain_val)
  RegField5/1 -> Gain_duc_input/7(carr4_gain_val)
  RegField6/1 -> Gain_duc_input/8(carr5_gain_val)
  RegField7/1 -> Gain_duc_input/9(carr6_gain_val)
  RegField8/1 -> Gain_duc_input/10(carr7_gain_val)
  RegField9/1 -> Gain_duc_input/11(carr8_gain_val)
  PipeReg_lduc_hduc1_L2/1 -> DUC_IN_PM/3("data "), Gain_duc_input/1(a)
  PipeReg_lduc_hduc1_L2/2 -> DUC_IN_PM/1(valid), Gain_duc_input/2(v)
  PipeReg_lduc_hduc1_L2/3 -> DUC_IN_PM/2(channel), Gain_duc_input/3(c)
  A1_valid/1 -> PipeReg_lduc_hduc1_L2/2, PipeReg_avln_avln_R/2
  A1_data/1 -> PipeReg_lduc_hduc1_L2/1, PipeReg_avln_avln_R/1
  A1_chan/1 -> PipeReg_lduc_hduc1_L2/3, PipeReg_avln_avln_R/3
  Gain_duc_input/2(gain_c_out) -> LDUC/2(In_c)
  Gain_duc_input/3(gain_real_out) -> LDUC/3(In_d)
  PipeReg_lduc_RC_R/1 -> DUC_SUMMER_PM/3("data "), Gain_summer/1(a)
  PipeReg_lduc_RC_R/2 -> DUC_SUMMER_PM/1(valid), Gain_summer/2(v)
  PipeReg_lduc_RC_R/3 -> DUC_SUMMER_PM/2(channel), Gain_summer/3(c)
  RegField10/1 -> Gain_summer/4(Ant1_gain_val)
  RegField11/1 -> Gain_summer/5(Antr2_gain_val)
  PipeReg_lduc_hduc1_L/1 -> PipeReg_lduc_hduc1_R/1
  PipeReg_lduc_hduc1_L/2 -> PipeReg_lduc_hduc1_R/2
  PipeReg_lduc_hduc1_L/3 -> PipeReg_lduc_hduc1_R/3
  Gain_summer/1(gain_real_out) -> PipeReg_lduc_hduc1_L/1
  Gain_summer/2(gain_v_out) -> PipeReg_lduc_hduc1_L/2
  Gain_summer/3(gain_c_out) -> PipeReg_lduc_hduc1_L/3
  RegField12/1 -> Gain_dpd_input/4(dpd1_gain_val)
  RegField13/1 -> Gain_dpd_input/5(dpd2_gain_val)
  PipeReg_HDCU2_RC_L1/1 -> PipeReg_HDCU2_RC1/1
  PipeReg_HDCU2_RC_L1/2 -> PipeReg_HDCU2_RC1/2
  PipeReg_HDCU2_RC_L1/3 -> PipeReg_HDCU2_RC1/3
  Gain_duc_input/1(gain_v_out) -> LDUC/1(In_v)
  LDUC/3(Out3) -> PipeReg_lduc_RC_L/3
  DPD/2(source_valid) -> DUC_DPD1_OUT_PM/1(valid), PipeReg_dpd1gain_dpd1clip_L/2
  DPD/4(source_data1) -> PipeReg_dpd2gain_dpd2clip_L/1, DUC_DPD2_OUT_PM/3("data ")
  DPD/5(source_valid1) -> DUC_DPD2_OUT_PM/1(valid), PipeReg_dpd2gain_dpd2clip_L/2
  DPD/3(source_channel) -> DUC_DPD1_OUT_PM/2(channel), PipeReg_dpd1gain_dpd1clip_L/3
  DPD/6(source_channel1) -> DUC_DPD2_OUT_PM/2(channel), PipeReg_dpd2gain_dpd2clip_L/3
  1ms_pulse/1 -> SampleDelay/1
  RegField/1 -> LDUC/5(sum_shift)
  SampleDelay/1 -> DUC_IN_PM/4(pulse_1msec), DUC_DPD1_OUT_PM/4(pulse_1msec), DUC_DPD2_OUT_PM/4(pulse_1msec), DUC_DPD_IN_PM/4(pulse_1msec), DUC_SUMMER_PM/4(pulse_1msec)
  PipeReg_dpd1gain_dpd1clip_L/1 -> PipeReg_dpd1gain_dpd1clip_R/1
  PipeReg_dpd1gain_dpd1clip_L/2 -> PipeReg_dpd1gain_dpd1clip_R/2
  PipeReg_dpd1gain_dpd1clip_L/3 -> PipeReg_dpd1gain_dpd1clip_R/3
  PipeReg_dpd2gain_dpd2clip_L/1 -> PipeReg_dpd2gain_dpd2clip_R/1
  PipeReg_dpd2gain_dpd2clip_L/2 -> PipeReg_dpd2gain_dpd2clip_R/2
  PipeReg_dpd2gain_dpd2clip_L/3 -> PipeReg_dpd2gain_dpd2clip_R/3
  PipeReg_dpd1gain_dpd1clip_R/1 -> DPD1_CLIPPER/1("data ")
  PipeReg_dpd1gain_dpd1clip_R/2 -> DPD1_CLIPPER/2(valid)
  PipeReg_dpd1gain_dpd1clip_R/3 -> DPD1_CLIPPER/3(channel)
  DPD1_CLIPPER/1(DATA_Out) -> PipeReg_dpd1clip_avln_L/1
  DPD1_CLIPPER/2(Valid_Out) -> PipeReg_dpd1clip_avln_L/2
  DPD1_CLIPPER/3(Chann_Out) -> PipeReg_dpd1clip_avln_L/3
  PipeReg_dpd1clip_avln_L/1 -> PipeReg_dpd1clip_avln_R/1
  PipeReg_dpd1clip_avln_L/2 -> PipeReg_dpd1clip_avln_R/2
  PipeReg_dpd1clip_avln_L/3 -> PipeReg_dpd1clip_avln_R/3
  PipeReg_dpd2clip_avln_L/1 -> PipeReg_dpd2clip_avln_R/1
  PipeReg_dpd2clip_avln_L/2 -> PipeReg_dpd2clip_avln_R/2
  PipeReg_dpd2clip_avln_L/3 -> PipeReg_dpd2clip_avln_R/3
  PipeReg_dpd2gain_dpd2clip_R/3 -> DPD2_CLIPPER/3(channel)
  PipeReg_dpd2gain_dpd2clip_R/2 -> DPD2_CLIPPER/2(valid)
  PipeReg_dpd2gain_dpd2clip_R/1 -> DPD2_CLIPPER/1("data ")
  DPD2_CLIPPER/1(DATA_Out) -> PipeReg_dpd2clip_avln_L/1
  DPD2_CLIPPER/2(Valid_Out) -> PipeReg_dpd2clip_avln_L/2
  DPD2_CLIPPER/3(Chann_Out) -> PipeReg_dpd2clip_avln_L/3
  RegField14/1 -> DPD2_CLIPPER/4(scale_bit)
  RegField1/1 -> DPD1_CLIPPER/4(scale_bit)
  PipeReg_2in1/3 -> PipeReg_2in/3
  PipeReg_2in1/4 -> PipeReg_2in/4
  PipeReg_2in1/1 -> PipeReg_2in/1
  PipeReg_2in1/2 -> PipeReg_2in/2
  DPD/1(source_data) -> DUC_DPD1_OUT_PM/3("data "), PipeReg_dpd1gain_dpd1clip_L/1
  Data Type Conversion2/1 -> Abs2/1
  Abs3/1 -> Scope1/2  "CFR OUTPUT"
  Abs2/1 -> Scope1/1  "CFR INPUT"
  Data Type Conversion4/1 -> Abs3/1
  HDUC_STG2/1(q1) -> PipeReg_HDCU2_RC_L1/1
  HDUC_STG2/2(qv) -> PipeReg_HDCU2_RC_L1/2
  HDUC_STG2/3(qc) -> PipeReg_HDCU2_RC_L1/3
  PipeReg_HDCU2_RC1/1 -> REAL_COMPLEX2/1(a1)
  PipeReg_HDCU2_RC1/2 -> REAL_COMPLEX2/2(v)
  PipeReg_HDCU2_RC1/3 -> REAL_COMPLEX2/3(c)
  PipeReg_2in/1 -> Mux/1
  PipeReg_2in/2 -> Mux/2
  Mux/1 -> COMPLEX_REAL/1(a1)
  PipeReg_2in/3 -> COMPLEX_REAL/2(v)
  PipeReg_2in/4 -> COMPLEX_REAL/3(c)
  COMPLEX_REAL/1(q1) -> DUC_DPD_IN_PM/3("data "), Gain_dpd_input/1(a)
  COMPLEX_REAL/2(q_v) -> DUC_DPD_IN_PM/1(valid), Gain_dpd_input/2(v)
  COMPLEX_REAL/3(q_c) -> DUC_DPD_IN_PM/2(channel), Gain_dpd_input/3(c)
  Gain_dpd_input/1(gain_real_out) -> REAL_COMPLEX1/1(a1)
  Gain_dpd_input/2(gain_v_out) -> REAL_COMPLEX1/2(v)
  Gain_dpd_input/3(gain_c_out) -> REAL_COMPLEX1/3(c)
  REAL_COMPLEX1/1(q1) -> Complex to Real-Imag/1, DPD/1(dpd_ant1_data)
  REAL_COMPLEX1/2(q2) -> DPD/2(dpd_ant2_data)
  REAL_COMPLEX1/3(q_v) -> DPD_ANT1_IN_valid/1, DPD/3(sink_valid)
  REAL_COMPLEX1/4(q_c) -> DPD_ANT1_IN_chan/1, DPD/4(sink_channel)
  RegBit/1 -> DUC_IN_PM/5(Reg_busy_bit), DUC_DPD1_OUT_PM/5(Reg_busy_bit), DUC_DPD2_OUT_PM/5(Reg_busy_bit), DUC_DPD_IN_PM/5(Reg_busy_bit), DUC_SUMMER_PM/5(Reg_busy_bit)
  Complex to Real-Imag1/1 -> BitCombine1/1
  Complex to Real-Imag1/2 -> BitCombine1/2
  PipeReg_HDUC2_RC_L1/1 -> Complex to Real-Imag1/1
  BLIND_CFR/1(q1) -> Data Type Conversion4/1, To Workspace3/1, PipeReg_HDUC2_RC_L1/1, PipeReg_2in1/1
  BLIND_CFR/2(q2) -> PipeReg_2in1/2
  BLIND_CFR/3(qv) -> PipeReg_HDUC2_RC_L1/2, PipeReg_2in1/3
  BLIND_CFR/4(qc) -> PipeReg_HDUC2_RC_L1/3, PipeReg_2in1/4
  REAL_COMPLEX2/1(q1) -> Data Type Conversion2/1, To Workspace1/1, BLIND_CFR/1(d1)
  REAL_COMPLEX2/4(q_c) -> BLIND_CFR/4(c)
  REAL_COMPLEX2/2(q2) -> BLIND_CFR/2(d2)
  REAL_COMPLEX2/3(q_v) -> BLIND_CFR/3(v)

== system downlink_4c2t/Subsystem ==
  Convert Input to Desired Datatype{1..8} (8 alike) : DataTypeConversion  OutDataTypeStr=fixdt(1,DUC_LINEUP_param.input_word_length,DUC_LINEUP_param.input_fraction_length)  SaturateOnIntegerOverflow=on
  Subsystem : Subsystem
  Test vector Generation Unit : Subsystem
  Out_valid : Outport
  Out_chan : Outport  Port=2
  Out_data : Outport  Port=3
  wires:
  Test vector Generation Unit/2(A1xC1_Valid) -> Subsystem/2(Carrier1_Valid)
  Test vector Generation Unit/3(A1xC1_Chan) -> Subsystem/3(Carrier1_Chann)
  Test vector Generation Unit/5(A1xC2_Valid) -> Subsystem/5(Carrier2_Valid)
  Test vector Generation Unit/6(A1xC2_Chan) -> Subsystem/6(Carrier2_Chann)
  Convert Input to Desired Datatype1/1 -> Subsystem/1(Carrier1_Data)
  Convert Input to Desired Datatype2/1 -> Subsystem/4(Carrier2_Data)
  Convert Input to Desired Datatype4/1 -> Subsystem/10(Carrier4_Data)
  Convert Input to Desired Datatype3/1 -> Subsystem/7(Carrier3_Data)
  Test vector Generation Unit/8(A1xC3_Valid) -> Subsystem/8(Carrier3_Valid)
  Test vector Generation Unit/9(A1xC3_Chan) -> Subsystem/9(Carrier3_Chann)
  Test vector Generation Unit/11(A1xC4_Valid) -> Subsystem/11(Carrier4_Valid)
  Test vector Generation Unit/12(A1xC4_Chan) -> Subsystem/12(Carrier4_Chann)
  Convert Input to Desired Datatype8/1 -> Subsystem/22(Carrier4_Data1)
  Convert Input to Desired Datatype7/1 -> Subsystem/19(Carrier3_Data1)
  Convert Input to Desired Datatype6/1 -> Subsystem/16(Carrier2_Data1)
  Convert Input to Desired Datatype5/1 -> Subsystem/13(Carrier1_Data1)
  Test vector Generation Unit/14(A2xC1_Valid) -> Subsystem/14(Carrier1_Valid1)
  Test vector Generation Unit/15(A2xC1_Chan) -> Subsystem/15(Carrier1_Chann1)
  Test vector Generation Unit/18(A2xC2_Chan) -> Subsystem/18(Carrier2_Chann1)
  Test vector Generation Unit/20(A2xC3_Valid) -> Subsystem/20(Carrier3_Valid1)
  Test vector Generation Unit/21(A2xC3_Chan) -> Subsystem/21(Carrier3_Chann1)
  Test vector Generation Unit/16(A2xC2_Data) -> Convert Input to Desired Datatype6/1
  Test vector Generation Unit/17(A2xC2_Valid) -> Subsystem/17(Carrier2_Valid1)
  Test vector Generation Unit/22(A2xC4_Data) -> Convert Input to Desired Datatype8/1
  Test vector Generation Unit/19(A2xC3_Data) -> Convert Input to Desired Datatype7/1
  Test vector Generation Unit/23(A2xC4_Valid) -> Subsystem/23(Carrier4_Valid1)
  Test vector Generation Unit/24(A2xC4_Chan) -> Subsystem/24(Carrier4_Chann1)
  Test vector Generation Unit/7(A1xC3_Data) -> Convert Input to Desired Datatype3/1
  Test vector Generation Unit/4(A1xC2_Data) -> Convert Input to Desired Datatype2/1
  Test vector Generation Unit/10(A1xC4_Data) -> Convert Input to Desired Datatype4/1
  Test vector Generation Unit/13(A2xC1_Data) -> Convert Input to Desired Datatype5/1
  Test vector Generation Unit/1(A1xC1_Data) -> Convert Input to Desired Datatype1/1
  Subsystem/2(Out_Valid) -> Out_valid/1
  Subsystem/3(Out_chan) -> Out_chan/1
  Subsystem/1(Out_data) -> Out_data/1

== system downlink_4c2t/DUT/ANT1_rfp ==
  GPOut : DSPBAPrim/GPOut  primtype=gpout  nInputs=evalAionMaskParam(gcb,'value',1)  nOutputs=evalAionMaskParam(gcb,'value',1)  omode=Inherit via internal rule  otype=sfix(16)  scale=2^-15  rndmethod=Unbiased  factor=1  satmethod=Symmetric  shift_vec=[0 1 2 -1]  value=1  inPortNames=[' ' ' ' ' ' ' ' ' ' ' ' ' ' ' ' ' ' ' ' ' ' ' ' ' ' ' ' ' ' ' ' ' ' ' ' ' ' ' ' ' ' ' ' ' ' ' ' ' ' ' ' ' ' ' ' ' ' ' ' ' ' ' ' ' ' ' ' ' ']'  outPortNames=[' ' ' ' ' ' ' ' ' ' ' ' ' ' ' ' ' ' ' ' ' ' ' ' ' ' ' ' ' ' ' ' ' ' ' ' ' ' ' ' ' ' ' ' ' ' ' ' ' ' ' ' ' ' ' ' ' ' ' ' ' ' ' ' ' ' ' ' ' ']'  dspbaimage=dspba_prim.jpg  text=fprintf('GPOut');  style=Optimised  visibilities=1024  latencyCorrection=0  version=20090407
  SynthesisInfo : DSPBAPrim/SynthesisInfo  primtype=synthinfo  nInputs=0  nOutputs=0  omode=Inherit via internal rule  otype=sfix(16)  scale=2^-15  rndmethod=Truncate  factor=1  satmethod=Symmetric  shift_vec=[0 1 2 -1]  value=99  inPortNames=[' '; ' ';]  outPortNames=[' ']  dspbaimage=dspba_prim_ctrl.jpg  text=fprintf('Style=%s', style);  style=Scheduled  visibilities=2^15+2^17+2^18+2^19  constraintInUse=off  constraintRelation=>  constraintLimit=2  bitAccurate=off  version=20150220
  zero_idx1 : DSPBAPrim/Const  primtype=const  nInputs=0  nOutputs=1  omode=boolean  otype=ufix(1)  scale=0  rndmethod=Unbiased  factor=1  satmethod=Symmetric  shift_vec=[0 1 2 -1]  value=1  inPortNames=['+'; '+';]  outPortNames=[' ']  dspbaimage=dspba_prim.jpg  text=fprintf('%s', num2str(value));  style=Optimised  visibilities=8 + 1024  floatPrecision=float32_m23  version=20120820
  Out_RFP : Outport
  wires:
  zero_idx1/1 -> GPOut/1
  GPOut/1 -> Out_RFP/1

== system downlink_4c2t/DUT/ANT2_rfp ==
  GPOut : DSPBAPrim/GPOut  primtype=gpout  nInputs=evalAionMaskParam(gcb,'value',1)  nOutputs=evalAionMaskParam(gcb,'value',1)  omode=Inherit via internal rule  otype=sfix(16)  scale=2^-15  rndmethod=Unbiased  factor=1  satmethod=Symmetric  shift_vec=[0 1 2 -1]  value=1  inPortNames=[' ' ' ' ' ' ' ' ' ' ' ' ' ' ' ' ' ' ' ' ' ' ' ' ' ' ' ' ' ' ' ' ' ' ' ' ' ' ' ' ' ' ' ' ' ' ' ' ' ' ' ' ' ' ' ' ' ' ' ' ' ' ' ' ' ' ' ' ' ']'  outPortNames=[' ' ' ' ' ' ' ' ' ' ' ' ' ' ' ' ' ' ' ' ' ' ' ' ' ' ' ' ' ' ' ' ' ' ' ' ' ' ' ' ' ' ' ' ' ' ' ' ' ' ' ' ' ' ' ' ' ' ' ' ' ' ' ' ' ' ' ' ' ']'  dspbaimage=dspba_prim.jpg  text=fprintf('GPOut');  style=Optimised  visibilities=1024  latencyCorrection=0  version=20090407
  SynthesisInfo : DSPBAPrim/SynthesisInfo  primtype=synthinfo  nInputs=0  nOutputs=0  omode=Inherit via internal rule  otype=sfix(16)  scale=2^-15  rndmethod=Truncate  factor=1  satmethod=Symmetric  shift_vec=[0 1 2 -1]  value=99  inPortNames=[' '; ' ';]  outPortNames=[' ']  dspbaimage=dspba_prim_ctrl.jpg  text=fprintf('Style=%s', style);  style=Scheduled  visibilities=2^15+2^17+2^18+2^19  constraintInUse=off  constraintRelation=>  constraintLimit=2  bitAccurate=off  version=20150220
  zero_idx1 : DSPBAPrim/Const  primtype=const  nInputs=0  nOutputs=1  omode=boolean  otype=ufix(1)  scale=0  rndmethod=Unbiased  factor=1  satmethod=Symmetric  shift_vec=[0 1 2 -1]  value=1  inPortNames=['+'; '+';]  outPortNames=[' ']  dspbaimage=dspba_prim.jpg  text=fprintf('%s', num2str(value));  style=Optimised  visibilities=8 + 1024  floatPrecision=float32_m23  version=20120820
  Out_RFP : Outport
  wires:
  GPOut/1 -> Out_RFP/1
  zero_idx1/1 -> GPOut/1

== system downlink_4c2t/DUT/BLIND_CFR ==
  d1 : Inport
  d2 : Inport  Port=2
  v : Inport  Port=3
  c : Inport  Port=4
  CFR1 : Subsystem  mask(Altera CFR Library Block){clk=clock_rate, block_id=cfr0_id, block_id_addr=REG_dut_id_addr, cfr_Params=cfr_Params0, REG=REG}
      mask prompts: clk "System clock"; block_id "Unique ID of CFR"; block_id_addr "CFR ID address"; cfr_Params "CFR Configuration Structure"; REG "Register Map"
      mask help:
      | The block has the following parameters:
      |
      | "system clock" - the clock rate CFR module runs.
      |
      | "sample rate" - input signal sampling rate.
      |
      | "Folding Factor" - the number of folding for the module time-sharing;
      | It takes integer values between 1 and floor(system clock / sample rate).
      |
      | "Unique ID of CFR" is a unique numerical integer identifier for the CFR
      | block, this is used once the block is in a larger system to confirm the
      | correct block is being accessed.
      |
      | "CFR ID address" this is the relative address of the "Unique ID of CFR"
      | typically this is zero (at the CFR base address).
      |
      | "CFR Configuration Structure" - an array structure containing the
      | configuration of the CFR block. The length of this parameter specifies the
      | number of CFR core iterations instantiated.
      |
      | "Register Map" a structure containing the register map for CFR block.
      |
      | The settings of the above are exemplified in the setup script of the
      | altera_cfr example design.
      mask init:
      | %setup_cfr_block(iters, Iter_Params, REG, block_id, block_id_addr);
      mask Display:
      | color('w');
      | image(imread('dspba_prim.jpg'));
      | fprintf('Blind \n Crest-factor \n Reduction \n');
      | port_label('input',1,'valid');port_label('input',2,'channel');port_label('input',3,'xr');
      | port_label('output',1,'v');port_label('output',2,'c');port_label('output',3,'zr');
  CFR2 : Subsystem  mask(Altera CFR Library Block){clk=clock_rate, block_id=cfr0_id, block_id_addr=REG_dut_id_addr, cfr_Params=cfr_Params1, REG=REG}
      mask prompts: clk "System clock"; block_id "Unique ID of CFR"; block_id_addr "CFR ID address"; cfr_Params "CFR Configuration Structure"; REG "Register Map"
      mask help:
      | The block has the following parameters:
      |
      | "system clock" - the clock rate CFR module runs.
      |
      | "sample rate" - input signal sampling rate.
      |
      | "Folding Factor" - the number of folding for the module time-sharing;
      | It takes integer values between 1 and floor(system clock / sample rate).
      |
      | "Unique ID of CFR" is a unique numerical integer identifier for the CFR
      | block, this is used once the block is in a larger system to confirm the
      | correct block is being accessed.
      |
      | "CFR ID address" this is the relative address of the "Unique ID of CFR"
      | typically this is zero (at the CFR base address).
      |
      | "CFR Configuration Structure" - an array structure containing the
      | configuration of the CFR block. The length of this parameter specifies the
      | number of CFR core iterations instantiated.
      |
      | "Register Map" a structure containing the register map for CFR block.
      |
      | The settings of the above are exemplified in the setup script of the
      | altera_cfr example design.
      mask init:
      | %setup_cfr_block(iters, Iter_Params, REG, block_id, block_id_addr);
      mask Display:
      | color('w');
      | image(imread('dspba_prim.jpg'));
      | fprintf('Blind \n Crest-factor \n Reduction \n');
      | port_label('input',1,'valid');port_label('input',2,'channel');port_label('input',3,'xr');
      | port_label('output',1,'v');port_label('output',2,'c');port_label('output',3,'zr');
  Terminator : Terminator
  Terminator1 : Terminator
  q1 : Outport
  q2 : Outport  Port=2
  qv : Outport  Port=3
  qc : Outport  Port=4
  wires:
  CFR2/3(Out3) -> q2/1
  c/1 -> CFR2/2(In2), CFR1/2(In2)
  d2/1 -> CFR2/3(In3)
  d1/1 -> CFR1/3(In3)
  CFR1/3(Out3) -> q1/1
  CFR1/2(Out2) -> qc/1
  v/1 -> CFR2/1(In1), CFR1/1(In1)
  CFR1/1(Out1) -> qv/1
  CFR2/1(Out1) -> Terminator/1
  CFR2/2(Out2) -> Terminator1/1
